simulink model "AttitudeDetermination"  (R2024b)
settings: Solver=VariableStepAuto  StartTime=0.0  StopTime=10.0  RelTol=1e-3
libraries: matrix_library x6
settings Model: Creator=filippocamaleonte  LastModifiedBy=filippocamaleonte

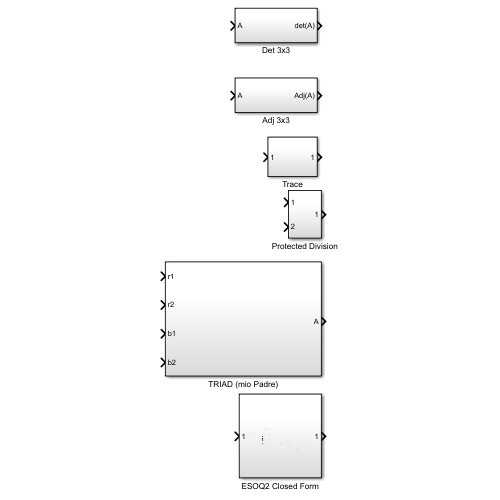
[thumbnail: Simulink's stored preview of the top-level diagram]
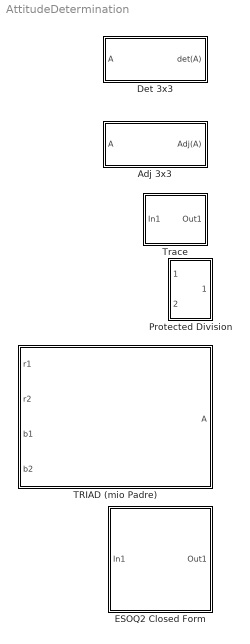
== system AttitudeDetermination ==
  Adj 3x3 : Subsystem
  Det 3x3 : Subsystem
  ESOQ2 Closed Form : Subsystem
  Protected Division : Subsystem
  TRIAD (mio Padre) : Subsystem
  Trace : Subsystem

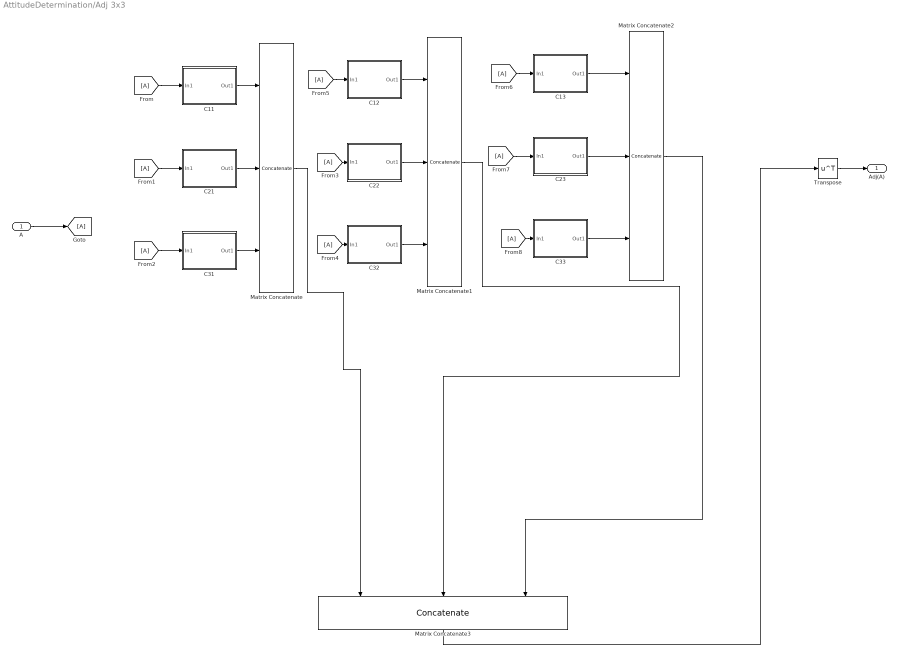
== system AttitudeDetermination/Adj 3x3 ==
  A : Inport
  C11 : Subsystem
  C12 : Subsystem
  C13 : Subsystem
  C21 : Subsystem
  C22 : Subsystem
  C23 : Subsystem
  C31 : Subsystem
  C32 : Subsystem
  C33 : Subsystem
  From{,1..8} (9 alike) : From
  Goto : Goto
  Matrix Concatenate : Concatenate  NumInputs=3  Mode=Multidimensional array
  Matrix Concatenate1 : Concatenate  NumInputs=3  Mode=Multidimensional array
  Matrix Concatenate2 : Concatenate  NumInputs=3  Mode=Multidimensional array
  Matrix Concatenate3 : Concatenate  NumInputs=3  Mode=Multidimensional array  ConcatenateDimension=2
  Transpose : Math  Operator=transpose
  Adj(A) : Outport
  wires:
  Transpose/1 -> Adj(A)/1
  A/1 -> Goto/1
  C11/1(Out1) -> Matrix Concatenate/1
  C21/1(Out1) -> Matrix Concatenate/2
  C31/1(Out1) -> Matrix Concatenate/3
  C22/1(Out1) -> Matrix Concatenate1/2
  C12/1(Out1) -> Matrix Concatenate1/1
  C32/1(Out1) -> Matrix Concatenate1/3
  C23/1(Out1) -> Matrix Concatenate2/2
  C13/1(Out1) -> Matrix Concatenate2/1
  C33/1(Out1) -> Matrix Concatenate2/3
  Matrix Concatenate3/1 -> Transpose/1
  Matrix Concatenate2/1 -> Matrix Concatenate3/3
  Matrix Concatenate1/1 -> Matrix Concatenate3/2
  Matrix Concatenate/1 -> Matrix Concatenate3/1
  From/1 -> C11/1(In1)
  From1/1 -> C21/1(In1)
  From2/1 -> C31/1(In1)
  From3/1 -> C22/1(In1)
  From4/1 -> C32/1(In1)
  From5/1 -> C12/1(In1)
  From6/1 -> C13/1(In1)
  From7/1 -> C23/1(In1)
  From8/1 -> C33/1(In1)

== system AttitudeDetermination/Det 3x3 ==
  A : Inport
  Adj 3x3 : Subsystem
  Matrix Multiply : Product  Multiplication=Matrix(*)
  Selector : Selector  NumberOfDimensions=2  InputPortWidth=3  IndexOptions=Index vector (dialog),Index vector (dialog)  Indices=1,1  OutputSizes=1,1
  det(A) : Outport
  wires:
  A/1 -> Adj 3x3/1(In1), Matrix Multiply/1
  Adj 3x3/1(Out1) -> Matrix Multiply/2
  Matrix Multiply/1 -> Selector/1
  Selector/1 -> det(A)/1

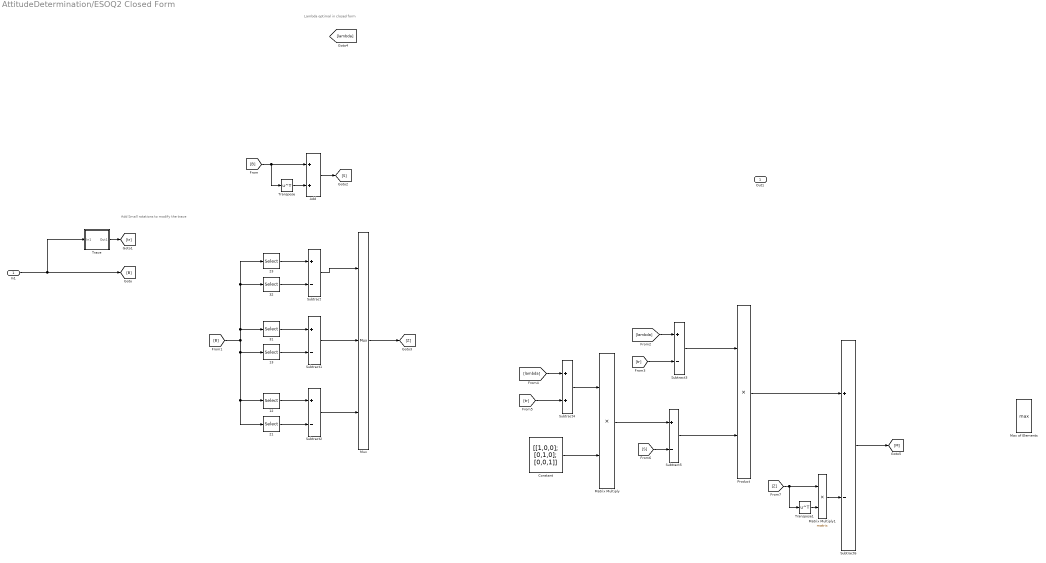
== system AttitudeDetermination/ESOQ2 Closed Form ==
  note: Lambda optimal in closed form
  note: Add Small rotations to modify the trace
  In1 : Inport
  12 : Selector  NumberOfDimensions=2  InputPortWidth=3  IndexOptions=Index vector (dialog),Index vector (dialog)  Indices=1,2  OutputSizes=1,1
  13 : Selector  NumberOfDimensions=2  InputPortWidth=3  IndexOptions=Index vector (dialog),Index vector (dialog)  Indices=1,3  OutputSizes=1,1
  21 : Selector  NumberOfDimensions=2  InputPortWidth=3  IndexOptions=Index vector (dialog),Index vector (dialog)  Indices=2,1  OutputSizes=1,1
  23 : Selector  NumberOfDimensions=2  InputPortWidth=3  IndexOptions=Index vector (dialog),Index vector (dialog)  Indices=2,3  OutputSizes=1,1
  31 : Selector  NumberOfDimensions=2  InputPortWidth=3  IndexOptions=Index vector (dialog),Index vector (dialog)  Indices=3,1  OutputSizes=1,1
  32 : Selector  NumberOfDimensions=2  InputPortWidth=3  IndexOptions=Index vector (dialog),Index vector (dialog)  Indices=3,2  OutputSizes=1,1
  Add : Sum
  Constant : Constant  Value=[[1,0,0]; [0,1,0]; [0,0,1]]
  Matrix Multiply : Product
  Matrix Multiply1 : Product  Multiplication=Matrix(*)
  Max of Elements : MinMax  Function=max
  Mux : Mux  Inputs=3
  Product : Product
  Subtract{,1..3,5..6} (6 alike) : Sum  Inputs=+-
  Subtract4 : Sum
  Trace : Subsystem
  Transpose : Math  Operator=transpose
  Transpose1 : Math  Operator=transpose
  Out1 : Outport
  wires:
  Trace/1(Out1) -> [tr]
  In1/1 -> Trace/1(In1), [B]
  [B] -> Transpose/1, Add/1
  Transpose/1 -> Add/2
  Add/1 -> [S]
  23/1 -> Subtract/1
  32/1 -> Subtract/2
  31/1 -> Subtract1/1
  21/1 -> Subtract2/2
  13/1 -> Subtract1/2
  12/1 -> Subtract2/1
  [B] -> 31/1, 32/1, 23/1, 13/1, 12/1, 21/1
  Subtract1/1 -> Mux/2
  Subtract/1 -> Mux/1
  Subtract2/1 -> Mux/3
  Mux/1 -> [Z]
  [lambda] -> Subtract3/1
  [tr] -> Subtract3/2
  [tr] -> Subtract4/2
  [lambda] -> Subtract4/1
  Subtract4/1 -> Matrix Multiply/1
  Constant/1 -> Matrix Multiply/2
  Matrix Multiply/1 -> Subtract5/1
  [S] -> Subtract5/2
  Product/1 -> Subtract6/1
  Subtract3/1 -> Product/1
  Subtract5/1 -> Product/2
  Matrix Multiply1/1 -> Subtract6/2
  [Z] -> Transpose1/1, Matrix Multiply1/1
  Transpose1/1 -> Matrix Multiply1/2
  Subtract6/1 -> [M]

== system AttitudeDetermination/Protected Division ==
  In1 : Inport
  In2 : Inport  Port=2
  Constant : Constant  Value=eps
  Divide : Product  Inputs=*/
  Switch : Switch  Criteria=u2 ~= 0  SaturateOnIntegerOverflow=off  InputSameDT=off
  Out1 : Outport
  wires:
  Divide/1 -> Out1/1
  In1/1 -> Divide/1
  In2/1 -> Switch/1, Switch/2
  Switch/1 -> Divide/2
  Constant/1 -> Switch/3

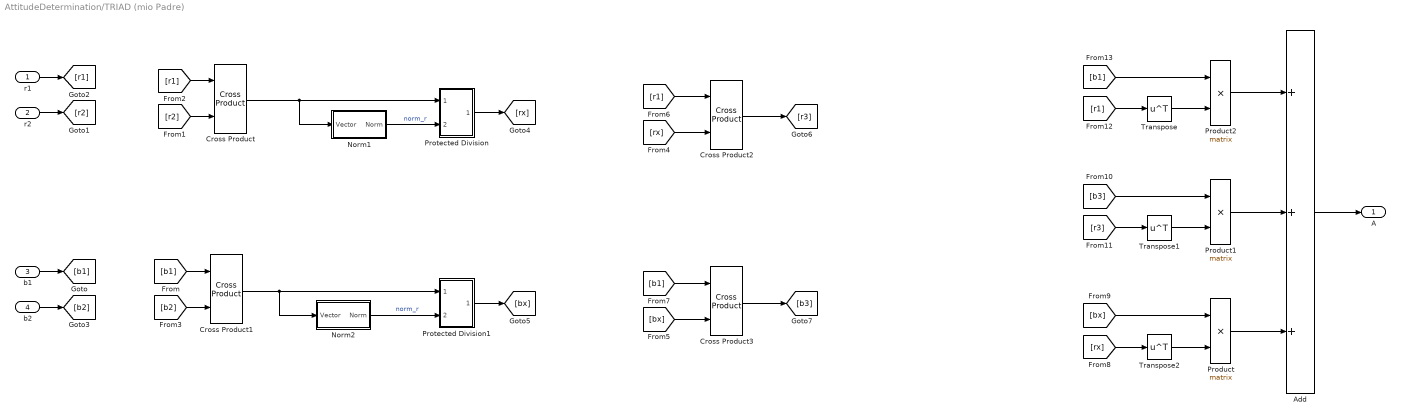
== system AttitudeDetermination/TRIAD (mio Padre) ==
  r1 : Inport
  r2 : Inport  Port=2
  b1 : Inport  Port=3
  b2 : Inport  Port=4
  Add : Sum  Inputs=+++
  Cross Product{,1..3} (4 alike) : matrix_library/Cross Product
  Norm1 : Subsystem
  Norm2 : Subsystem
  Product : Product  Multiplication=Matrix(*)
  Product1 : Product  Multiplication=Matrix(*)
  Product2 : Product  Multiplication=Matrix(*)
  Protected Division : Subsystem
  Protected Division1 : Subsystem
  Transpose : Math  Operator=transpose
  Transpose1 : Math  Operator=transpose
  Transpose2 : Math  Operator=transpose
  A : Outport
  wires:
  Cross Product/1 -> Norm1/1(Vector), Protected Division/1(In1)
  Cross Product1/1 -> Norm2/1(Vector), Protected Division1/1(In1)
  b1/1 -> [b1]
  [b1] -> Cross Product1/1
  r2/1 -> [r2]
  [r2] -> Cross Product/2
  r1/1 -> [r1]
  [r1] -> Cross Product/1
  b2/1 -> [b2]
  [b2] -> Cross Product1/2
  Norm1/1(Norm) -> Protected Division/2(Norm)  "norm_r"
  Norm2/1(Norm) -> Protected Division1/2(Norm)  "norm_r"
  Protected Division/1(Out1) -> [rx]
  Protected Division1/1(Out1) -> [bx]
  [rx] -> Cross Product2/2
  [bx] -> Cross Product3/2
  [r1] -> Cross Product2/1
  [b1] -> Cross Product3/1
  Cross Product2/1 -> [r3]
  Cross Product3/1 -> [b3]
  Add/1 -> A/1
  Product/1 -> Add/3
  Product1/1 -> Add/2
  Product2/1 -> Add/1
  Transpose/1 -> Product2/2
  Transpose1/1 -> Product1/2
  Transpose2/1 -> Product/2
  [rx] -> Transpose2/1
  [bx] -> Product/1
  [b3] -> Product1/1
  [r3] -> Transpose1/1
  [r1] -> Transpose/1
  [b1] -> Product2/1

== system AttitudeDetermination/Trace ==
  In1 : Inport
  Extract Diagonal : matrix_library/Extract Diagonal
      settings: LibrarySourceBlock=|
      | simulink/Matrix
      | Operations/Extract Diagonal
  Sum of Elements : Sum  Inputs=+
  Out1 : Outport
  wires:
  In1/1 -> Extract Diagonal/1
  Extract Diagonal/1 -> Sum of Elements/1
  Sum of Elements/1 -> Out1/1

== system AttitudeDetermination/Adj 3x3/C11 ==
  In1 : Inport
  22 : Selector  NumberOfDimensions=2  InputPortWidth=3  IndexOptions=Index vector (dialog),Index vector (dialog)  Indices=2,2  OutputSizes=1,1
  23 : Selector  NumberOfDimensions=2  InputPortWidth=3  IndexOptions=Index vector (dialog),Index vector (dialog)  Indices=2,3  OutputSizes=1,1
  32 : Selector  NumberOfDimensions=2  InputPortWidth=3  IndexOptions=Index vector (dialog),Index vector (dialog)  Indices=3,2  OutputSizes=1,1
  33 : Selector  NumberOfDimensions=2  InputPortWidth=3  IndexOptions=Index vector (dialog),Index vector (dialog)  Indices=3,3  OutputSizes=1,1
  Product : Product
  Product1 : Product
  Subtract : Sum  Inputs=+-
  Out1 : Outport
  wires:
  In1/1 -> 32/1, 23/1, 33/1, 22/1
  22/1 -> Product/1
  33/1 -> Product/2
  23/1 -> Product1/1
  32/1 -> Product1/2
  Subtract/1 -> Out1/1
  Product/1 -> Subtract/1
  Product1/1 -> Subtract/2

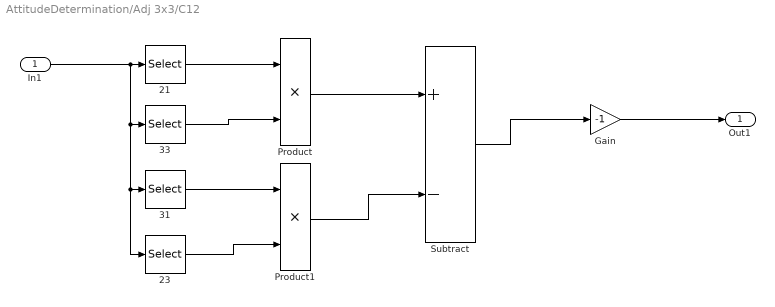
== system AttitudeDetermination/Adj 3x3/C12 ==
  In1 : Inport
  21 : Selector  NumberOfDimensions=2  InputPortWidth=3  IndexOptions=Index vector (dialog),Index vector (dialog)  Indices=2,1  OutputSizes=1,1
  23 : Selector  NumberOfDimensions=2  InputPortWidth=3  IndexOptions=Index vector (dialog),Index vector (dialog)  Indices=2,3  OutputSizes=1,1
  31 : Selector  NumberOfDimensions=2  InputPortWidth=3  IndexOptions=Index vector (dialog),Index vector (dialog)  Indices=3,1  OutputSizes=1,1
  33 : Selector  NumberOfDimensions=2  InputPortWidth=3  IndexOptions=Index vector (dialog),Index vector (dialog)  Indices=3,3  OutputSizes=1,1
  Gain : Gain  Gain=-1
  Product : Product
  Product1 : Product
  Subtract : Sum  Inputs=+-
  Out1 : Outport
  wires:
  In1/1 -> 23/1, 31/1, 33/1, 21/1
  21/1 -> Product/1
  33/1 -> Product/2
  31/1 -> Product1/1
  23/1 -> Product1/2
  Subtract/1 -> Gain/1
  Product/1 -> Subtract/1
  Product1/1 -> Subtract/2
  Gain/1 -> Out1/1

== system AttitudeDetermination/Adj 3x3/C13 ==
  In1 : Inport
  21 : Selector  NumberOfDimensions=2  InputPortWidth=3  IndexOptions=Index vector (dialog),Index vector (dialog)  Indices=2,1  OutputSizes=1,1
  22 : Selector  NumberOfDimensions=2  InputPortWidth=3  IndexOptions=Index vector (dialog),Index vector (dialog)  Indices=2,2  OutputSizes=1,1
  31 : Selector  NumberOfDimensions=2  InputPortWidth=3  IndexOptions=Index vector (dialog),Index vector (dialog)  Indices=3,1  OutputSizes=1,1
  32 : Selector  NumberOfDimensions=2  InputPortWidth=3  IndexOptions=Index vector (dialog),Index vector (dialog)  Indices=3,2  OutputSizes=1,1
  Product : Product
  Product1 : Product
  Subtract : Sum  Inputs=+-
  Out1 : Outport
  wires:
  In1/1 -> 31/1, 22/1, 32/1, 21/1
  21/1 -> Product/1
  32/1 -> Product/2
  22/1 -> Product1/1
  31/1 -> Product1/2
  Subtract/1 -> Out1/1
  Product/1 -> Subtract/1
  Product1/1 -> Subtract/2

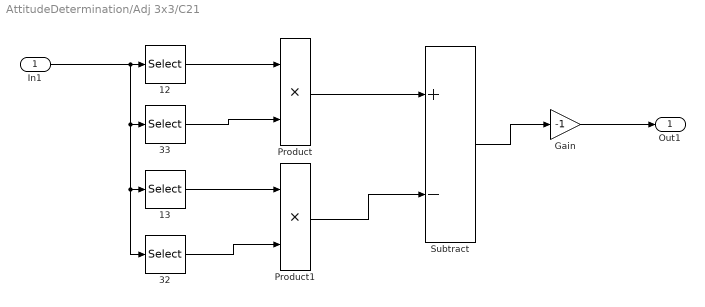
== system AttitudeDetermination/Adj 3x3/C21 ==
  In1 : Inport
  12 : Selector  NumberOfDimensions=2  InputPortWidth=3  IndexOptions=Index vector (dialog),Index vector (dialog)  Indices=1,2  OutputSizes=1,1
  13 : Selector  NumberOfDimensions=2  InputPortWidth=3  IndexOptions=Index vector (dialog),Index vector (dialog)  Indices=1,3  OutputSizes=1,1
  32 : Selector  NumberOfDimensions=2  InputPortWidth=3  IndexOptions=Index vector (dialog),Index vector (dialog)  Indices=3,2  OutputSizes=1,1
  33 : Selector  NumberOfDimensions=2  InputPortWidth=3  IndexOptions=Index vector (dialog),Index vector (dialog)  Indices=3,3  OutputSizes=1,1
  Gain : Gain  Gain=-1
  Product : Product
  Product1 : Product
  Subtract : Sum  Inputs=+-
  Out1 : Outport
  wires:
  In1/1 -> 32/1, 13/1, 33/1, 12/1
  12/1 -> Product/1
  33/1 -> Product/2
  13/1 -> Product1/1
  32/1 -> Product1/2
  Subtract/1 -> Gain/1
  Product/1 -> Subtract/1
  Product1/1 -> Subtract/2
  Gain/1 -> Out1/1

== system AttitudeDetermination/Adj 3x3/C22 ==
  In1 : Inport
  11 : Selector  NumberOfDimensions=2  InputPortWidth=3  IndexOptions=Index vector (dialog),Index vector (dialog)  Indices=1,1  OutputSizes=1,1
  13 : Selector  NumberOfDimensions=2  InputPortWidth=3  IndexOptions=Index vector (dialog),Index vector (dialog)  Indices=1,3  OutputSizes=1,1
  31 : Selector  NumberOfDimensions=2  InputPortWidth=3  IndexOptions=Index vector (dialog),Index vector (dialog)  Indices=3,1  OutputSizes=1,1
  33 : Selector  NumberOfDimensions=2  InputPortWidth=3  IndexOptions=Index vector (dialog),Index vector (dialog)  Indices=3,3  OutputSizes=1,1
  Product : Product
  Product1 : Product
  Subtract : Sum  Inputs=+-
  Out1 : Outport
  wires:
  In1/1 -> 31/1, 13/1, 33/1, 11/1
  11/1 -> Product/1
  33/1 -> Product/2
  13/1 -> Product1/1
  31/1 -> Product1/2
  Subtract/1 -> Out1/1
  Product/1 -> Subtract/1
  Product1/1 -> Subtract/2

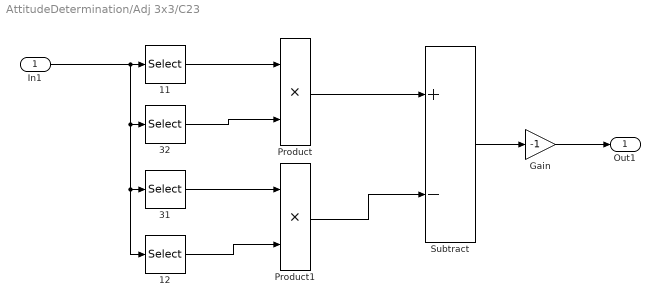
== system AttitudeDetermination/Adj 3x3/C23 ==
  In1 : Inport
  11 : Selector  NumberOfDimensions=2  InputPortWidth=3  IndexOptions=Index vector (dialog),Index vector (dialog)  Indices=1,1  OutputSizes=1,1
  12 : Selector  NumberOfDimensions=2  InputPortWidth=3  IndexOptions=Index vector (dialog),Index vector (dialog)  Indices=1,2  OutputSizes=1,1
  31 : Selector  NumberOfDimensions=2  InputPortWidth=3  IndexOptions=Index vector (dialog),Index vector (dialog)  Indices=3,1  OutputSizes=1,1
  32 : Selector  NumberOfDimensions=2  InputPortWidth=3  IndexOptions=Index vector (dialog),Index vector (dialog)  Indices=3,2  OutputSizes=1,1
  Gain : Gain  Gain=-1
  Product : Product
  Product1 : Product
  Subtract : Sum  Inputs=+-
  Out1 : Outport
  wires:
  In1/1 -> 12/1, 31/1, 32/1, 11/1
  11/1 -> Product/1
  32/1 -> Product/2
  31/1 -> Product1/1
  12/1 -> Product1/2
  Subtract/1 -> Gain/1
  Product/1 -> Subtract/1
  Product1/1 -> Subtract/2
  Gain/1 -> Out1/1

== system AttitudeDetermination/Adj 3x3/C31 ==
  In1 : Inport
  12 : Selector  NumberOfDimensions=2  InputPortWidth=3  IndexOptions=Index vector (dialog),Index vector (dialog)  Indices=1,2  OutputSizes=1,1
  13 : Selector  NumberOfDimensions=2  InputPortWidth=3  IndexOptions=Index vector (dialog),Index vector (dialog)  Indices=1,3  OutputSizes=1,1
  22 : Selector  NumberOfDimensions=2  InputPortWidth=3  IndexOptions=Index vector (dialog),Index vector (dialog)  Indices=2,2  OutputSizes=1,1
  23 : Selector  NumberOfDimensions=2  InputPortWidth=3  IndexOptions=Index vector (dialog),Index vector (dialog)  Indices=2,3  OutputSizes=1,1
  Product : Product
  Product1 : Product
  Subtract : Sum  Inputs=+-
  Out1 : Outport
  wires:
  In1/1 -> 22/1, 13/1, 23/1, 12/1
  12/1 -> Product/1
  23/1 -> Product/2
  13/1 -> Product1/1
  22/1 -> Product1/2
  Subtract/1 -> Out1/1
  Product/1 -> Subtract/1
  Product1/1 -> Subtract/2

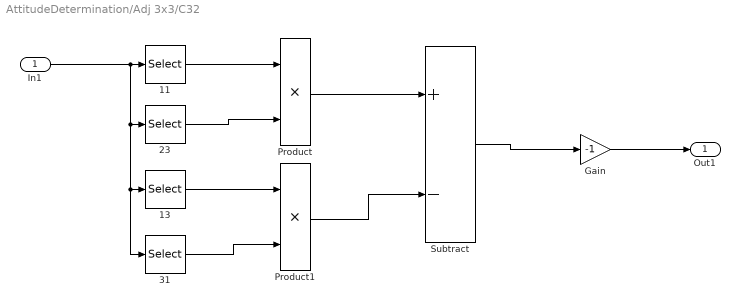
== system AttitudeDetermination/Adj 3x3/C32 ==
  In1 : Inport
  11 : Selector  NumberOfDimensions=2  InputPortWidth=3  IndexOptions=Index vector (dialog),Index vector (dialog)  Indices=1,1  OutputSizes=1,1
  13 : Selector  NumberOfDimensions=2  InputPortWidth=3  IndexOptions=Index vector (dialog),Index vector (dialog)  Indices=1,3  OutputSizes=1,1
  23 : Selector  NumberOfDimensions=2  InputPortWidth=3  IndexOptions=Index vector (dialog),Index vector (dialog)  Indices=2,3  OutputSizes=1,1
  31 : Selector  NumberOfDimensions=2  InputPortWidth=3  IndexOptions=Index vector (dialog),Index vector (dialog)  Indices=3,1  OutputSizes=1,1
  Gain : Gain  Gain=-1
  Product : Product
  Product1 : Product
  Subtract : Sum  Inputs=+-
  Out1 : Outport
  wires:
  In1/1 -> 31/1, 13/1, 23/1, 11/1
  11/1 -> Product/1
  23/1 -> Product/2
  13/1 -> Product1/1
  31/1 -> Product1/2
  Subtract/1 -> Gain/1
  Product/1 -> Subtract/1
  Product1/1 -> Subtract/2
  Gain/1 -> Out1/1

== system AttitudeDetermination/Adj 3x3/C33 ==
  In1 : Inport
  11 : Selector  NumberOfDimensions=2  InputPortWidth=3  IndexOptions=Index vector (dialog),Index vector (dialog)  Indices=1,1  OutputSizes=1,1
  12 : Selector  NumberOfDimensions=2  InputPortWidth=3  IndexOptions=Index vector (dialog),Index vector (dialog)  Indices=1,2  OutputSizes=1,1
  21 : Selector  NumberOfDimensions=2  InputPortWidth=3  IndexOptions=Index vector (dialog),Index vector (dialog)  Indices=2,1  OutputSizes=1,1
  22 : Selector  NumberOfDimensions=2  InputPortWidth=3  IndexOptions=Index vector (dialog),Index vector (dialog)  Indices=2,2  OutputSizes=1,1
  Product : Product
  Product1 : Product
  Subtract : Sum  Inputs=+-
  Out1 : Outport
  wires:
  In1/1 -> 21/1, 12/1, 22/1, 11/1
  11/1 -> Product/1
  22/1 -> Product/2
  12/1 -> Product1/1
  21/1 -> Product1/2
  Subtract/1 -> Out1/1
  Product/1 -> Subtract/1
  Product1/1 -> Subtract/2

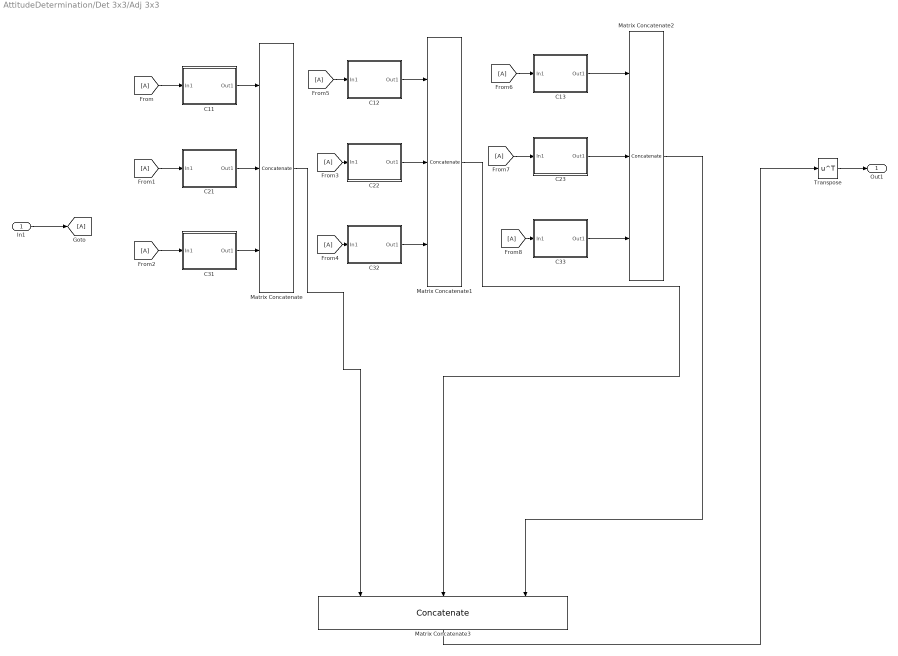
== system AttitudeDetermination/Det 3x3/Adj 3x3 ==
  In1 : Inport
  C11 : Subsystem
  C12 : Subsystem
  C13 : Subsystem
  C21 : Subsystem
  C22 : Subsystem
  C23 : Subsystem
  C31 : Subsystem
  C32 : Subsystem
  C33 : Subsystem
  From{,1..8} (9 alike) : From
  Goto : Goto
  Matrix Concatenate : Concatenate  NumInputs=3  Mode=Multidimensional array
  Matrix Concatenate1 : Concatenate  NumInputs=3  Mode=Multidimensional array
  Matrix Concatenate2 : Concatenate  NumInputs=3  Mode=Multidimensional array
  Matrix Concatenate3 : Concatenate  NumInputs=3  Mode=Multidimensional array  ConcatenateDimension=2
  Transpose : Math  Operator=transpose
  Out1 : Outport
  wires:
  Transpose/1 -> Out1/1
  In1/1 -> Goto/1
  C11/1(Out1) -> Matrix Concatenate/1
  C21/1(Out1) -> Matrix Concatenate/2
  C31/1(Out1) -> Matrix Concatenate/3
  C22/1(Out1) -> Matrix Concatenate1/2
  C12/1(Out1) -> Matrix Concatenate1/1
  C32/1(Out1) -> Matrix Concatenate1/3
  C23/1(Out1) -> Matrix Concatenate2/2
  C13/1(Out1) -> Matrix Concatenate2/1
  C33/1(Out1) -> Matrix Concatenate2/3
  Matrix Concatenate3/1 -> Transpose/1
  Matrix Concatenate2/1 -> Matrix Concatenate3/3
  Matrix Concatenate1/1 -> Matrix Concatenate3/2
  Matrix Concatenate/1 -> Matrix Concatenate3/1
  From/1 -> C11/1(In1)
  From1/1 -> C21/1(In1)
  From2/1 -> C31/1(In1)
  From3/1 -> C22/1(In1)
  From4/1 -> C32/1(In1)
  From5/1 -> C12/1(In1)
  From6/1 -> C13/1(In1)
  From7/1 -> C23/1(In1)
  From8/1 -> C33/1(In1)

== system AttitudeDetermination/ESOQ2 Closed Form/Trace ==
  In1 : Inport
  Extract Diagonal : matrix_library/Extract Diagonal
  Sum of Elements : Sum  Inputs=+
  Out1 : Outport
  wires:
  In1/1 -> Extract Diagonal/1
  Extract Diagonal/1 -> Sum of Elements/1
  Sum of Elements/1 -> Out1/1

== system AttitudeDetermination/TRIAD (mio Padre)/Norm1 ==
  Vector : Inport
  Add : Sum  Inputs=+++
  Demux : Demux  Outputs=3
  Sqrt : Sqrt
  Square : Math  Operator=square
  Square1 : Math  Operator=square
  Square2 : Math  Operator=square
  Norm : Outport
  wires:
  Square/1 -> Add/1
  Add/1 -> Sqrt/1
  Demux/3 -> Square1/1
  Square2/1 -> Add/2
  Square1/1 -> Add/3
  Demux/1 -> Square/1
  Demux/2 -> Square2/1
  Vector/1 -> Demux/1
  Sqrt/1 -> Norm/1

== system AttitudeDetermination/TRIAD (mio Padre)/Norm2 ==
  Vector : Inport
  Add : Sum  Inputs=+++
  Demux : Demux  Outputs=3
  Sqrt : Sqrt
  Square : Math  Operator=square
  Square1 : Math  Operator=square
  Square2 : Math  Operator=square
  Norm : Outport
  wires:
  Square/1 -> Add/1
  Add/1 -> Sqrt/1
  Demux/3 -> Square1/1
  Square2/1 -> Add/2
  Square1/1 -> Add/3
  Demux/1 -> Square/1
  Demux/2 -> Square2/1
  Vector/1 -> Demux/1
  Sqrt/1 -> Norm/1

== system AttitudeDetermination/TRIAD (mio Padre)/Protected Division ==
  In1 : Inport
  Norm : Inport  Port=2
  Constant : Constant  Value=eps
  Divide : Product  Inputs=*/
  Switch : Switch  Criteria=u2 ~= 0  SaturateOnIntegerOverflow=off  InputSameDT=off
  Out1 : Outport
  wires:
  Divide/1 -> Out1/1
  In1/1 -> Divide/1
  Norm/1 -> Switch/1, Switch/2
  Switch/1 -> Divide/2
  Constant/1 -> Switch/3

== system AttitudeDetermination/TRIAD (mio Padre)/Protected Division1 ==
  In1 : Inport
  Norm : Inport  Port=2
  Constant : Constant  Value=eps
  Divide : Product  Inputs=*/
  Switch : Switch  Criteria=u2 ~= 0  SaturateOnIntegerOverflow=off  InputSameDT=off
  Out1 : Outport
  wires:
  Divide/1 -> Out1/1
  In1/1 -> Divide/1
  Norm/1 -> Switch/1, Switch/2
  Switch/1 -> Divide/2
  Constant/1 -> Switch/3

== system AttitudeDetermination/Det 3x3/Adj 3x3/C11 ==
  In1 : Inport
  22 : Selector  NumberOfDimensions=2  InputPortWidth=3  IndexOptions=Index vector (dialog),Index vector (dialog)  Indices=2,2  OutputSizes=1,1
  23 : Selector  NumberOfDimensions=2  InputPortWidth=3  IndexOptions=Index vector (dialog),Index vector (dialog)  Indices=2,3  OutputSizes=1,1
  32 : Selector  NumberOfDimensions=2  InputPortWidth=3  IndexOptions=Index vector (dialog),Index vector (dialog)  Indices=3,2  OutputSizes=1,1
  33 : Selector  NumberOfDimensions=2  InputPortWidth=3  IndexOptions=Index vector (dialog),Index vector (dialog)  Indices=3,3  OutputSizes=1,1
  Product : Product
  Product1 : Product
  Subtract : Sum  Inputs=+-
  Out1 : Outport
  wires:
  In1/1 -> 32/1, 23/1, 33/1, 22/1
  22/1 -> Product/1
  33/1 -> Product/2
  23/1 -> Product1/1
  32/1 -> Product1/2
  Subtract/1 -> Out1/1
  Product/1 -> Subtract/1
  Product1/1 -> Subtract/2

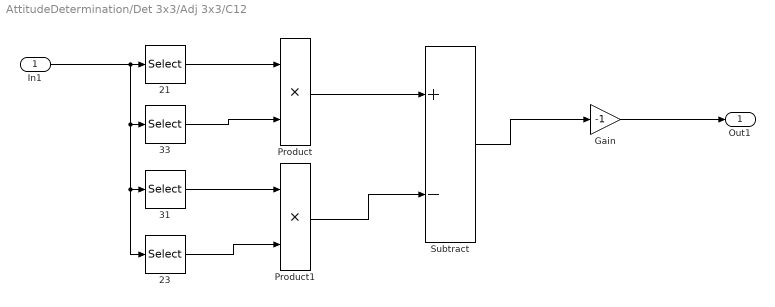
== system AttitudeDetermination/Det 3x3/Adj 3x3/C12 ==
  In1 : Inport
  21 : Selector  NumberOfDimensions=2  InputPortWidth=3  IndexOptions=Index vector (dialog),Index vector (dialog)  Indices=2,1  OutputSizes=1,1
  23 : Selector  NumberOfDimensions=2  InputPortWidth=3  IndexOptions=Index vector (dialog),Index vector (dialog)  Indices=2,3  OutputSizes=1,1
  31 : Selector  NumberOfDimensions=2  InputPortWidth=3  IndexOptions=Index vector (dialog),Index vector (dialog)  Indices=3,1  OutputSizes=1,1
  33 : Selector  NumberOfDimensions=2  InputPortWidth=3  IndexOptions=Index vector (dialog),Index vector (dialog)  Indices=3,3  OutputSizes=1,1
  Gain : Gain  Gain=-1
  Product : Product
  Product1 : Product
  Subtract : Sum  Inputs=+-
  Out1 : Outport
  wires:
  In1/1 -> 23/1, 31/1, 33/1, 21/1
  21/1 -> Product/1
  33/1 -> Product/2
  31/1 -> Product1/1
  23/1 -> Product1/2
  Subtract/1 -> Gain/1
  Product/1 -> Subtract/1
  Product1/1 -> Subtract/2
  Gain/1 -> Out1/1

== system AttitudeDetermination/Det 3x3/Adj 3x3/C13 ==
  In1 : Inport
  21 : Selector  NumberOfDimensions=2  InputPortWidth=3  IndexOptions=Index vector (dialog),Index vector (dialog)  Indices=2,1  OutputSizes=1,1
  22 : Selector  NumberOfDimensions=2  InputPortWidth=3  IndexOptions=Index vector (dialog),Index vector (dialog)  Indices=2,2  OutputSizes=1,1
  31 : Selector  NumberOfDimensions=2  InputPortWidth=3  IndexOptions=Index vector (dialog),Index vector (dialog)  Indices=3,1  OutputSizes=1,1
  32 : Selector  NumberOfDimensions=2  InputPortWidth=3  IndexOptions=Index vector (dialog),Index vector (dialog)  Indices=3,2  OutputSizes=1,1
  Product : Product
  Product1 : Product
  Subtract : Sum  Inputs=+-
  Out1 : Outport
  wires:
  In1/1 -> 31/1, 22/1, 32/1, 21/1
  21/1 -> Product/1
  32/1 -> Product/2
  22/1 -> Product1/1
  31/1 -> Product1/2
  Subtract/1 -> Out1/1
  Product/1 -> Subtract/1
  Product1/1 -> Subtract/2

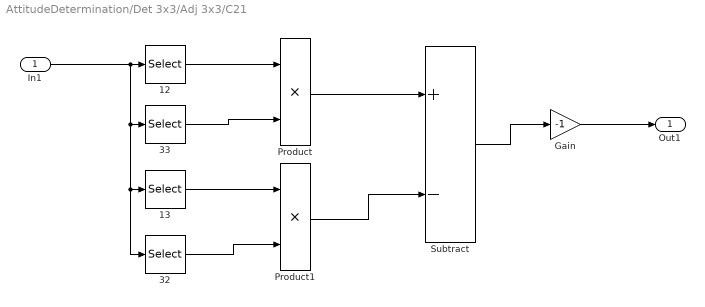
== system AttitudeDetermination/Det 3x3/Adj 3x3/C21 ==
  In1 : Inport
  12 : Selector  NumberOfDimensions=2  InputPortWidth=3  IndexOptions=Index vector (dialog),Index vector (dialog)  Indices=1,2  OutputSizes=1,1
  13 : Selector  NumberOfDimensions=2  InputPortWidth=3  IndexOptions=Index vector (dialog),Index vector (dialog)  Indices=1,3  OutputSizes=1,1
  32 : Selector  NumberOfDimensions=2  InputPortWidth=3  IndexOptions=Index vector (dialog),Index vector (dialog)  Indices=3,2  OutputSizes=1,1
  33 : Selector  NumberOfDimensions=2  InputPortWidth=3  IndexOptions=Index vector (dialog),Index vector (dialog)  Indices=3,3  OutputSizes=1,1
  Gain : Gain  Gain=-1
  Product : Product
  Product1 : Product
  Subtract : Sum  Inputs=+-
  Out1 : Outport
  wires:
  In1/1 -> 32/1, 13/1, 33/1, 12/1
  12/1 -> Product/1
  33/1 -> Product/2
  13/1 -> Product1/1
  32/1 -> Product1/2
  Subtract/1 -> Gain/1
  Product/1 -> Subtract/1
  Product1/1 -> Subtract/2
  Gain/1 -> Out1/1

== system AttitudeDetermination/Det 3x3/Adj 3x3/C22 ==
  In1 : Inport
  11 : Selector  NumberOfDimensions=2  InputPortWidth=3  IndexOptions=Index vector (dialog),Index vector (dialog)  Indices=1,1  OutputSizes=1,1
  13 : Selector  NumberOfDimensions=2  InputPortWidth=3  IndexOptions=Index vector (dialog),Index vector (dialog)  Indices=1,3  OutputSizes=1,1
  31 : Selector  NumberOfDimensions=2  InputPortWidth=3  IndexOptions=Index vector (dialog),Index vector (dialog)  Indices=3,1  OutputSizes=1,1
  33 : Selector  NumberOfDimensions=2  InputPortWidth=3  IndexOptions=Index vector (dialog),Index vector (dialog)  Indices=3,3  OutputSizes=1,1
  Product : Product
  Product1 : Product
  Subtract : Sum  Inputs=+-
  Out1 : Outport
  wires:
  In1/1 -> 31/1, 13/1, 33/1, 11/1
  11/1 -> Product/1
  33/1 -> Product/2
  13/1 -> Product1/1
  31/1 -> Product1/2
  Subtract/1 -> Out1/1
  Product/1 -> Subtract/1
  Product1/1 -> Subtract/2

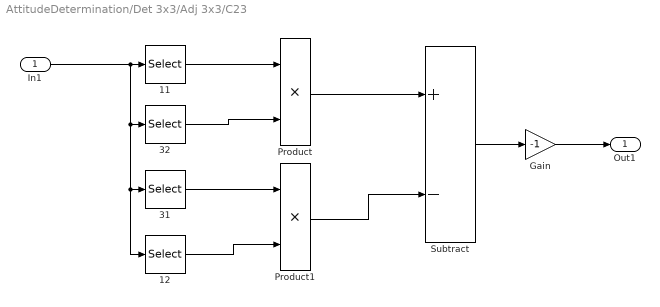
== system AttitudeDetermination/Det 3x3/Adj 3x3/C23 ==
  In1 : Inport
  11 : Selector  NumberOfDimensions=2  InputPortWidth=3  IndexOptions=Index vector (dialog),Index vector (dialog)  Indices=1,1  OutputSizes=1,1
  12 : Selector  NumberOfDimensions=2  InputPortWidth=3  IndexOptions=Index vector (dialog),Index vector (dialog)  Indices=1,2  OutputSizes=1,1
  31 : Selector  NumberOfDimensions=2  InputPortWidth=3  IndexOptions=Index vector (dialog),Index vector (dialog)  Indices=3,1  OutputSizes=1,1
  32 : Selector  NumberOfDimensions=2  InputPortWidth=3  IndexOptions=Index vector (dialog),Index vector (dialog)  Indices=3,2  OutputSizes=1,1
  Gain : Gain  Gain=-1
  Product : Product
  Product1 : Product
  Subtract : Sum  Inputs=+-
  Out1 : Outport
  wires:
  In1/1 -> 12/1, 31/1, 32/1, 11/1
  11/1 -> Product/1
  32/1 -> Product/2
  31/1 -> Product1/1
  12/1 -> Product1/2
  Subtract/1 -> Gain/1
  Product/1 -> Subtract/1
  Product1/1 -> Subtract/2
  Gain/1 -> Out1/1

== system AttitudeDetermination/Det 3x3/Adj 3x3/C31 ==
  In1 : Inport
  12 : Selector  NumberOfDimensions=2  InputPortWidth=3  IndexOptions=Index vector (dialog),Index vector (dialog)  Indices=1,2  OutputSizes=1,1
  13 : Selector  NumberOfDimensions=2  InputPortWidth=3  IndexOptions=Index vector (dialog),Index vector (dialog)  Indices=1,3  OutputSizes=1,1
  22 : Selector  NumberOfDimensions=2  InputPortWidth=3  IndexOptions=Index vector (dialog),Index vector (dialog)  Indices=2,2  OutputSizes=1,1
  23 : Selector  NumberOfDimensions=2  InputPortWidth=3  IndexOptions=Index vector (dialog),Index vector (dialog)  Indices=2,3  OutputSizes=1,1
  Product : Product
  Product1 : Product
  Subtract : Sum  Inputs=+-
  Out1 : Outport
  wires:
  In1/1 -> 22/1, 13/1, 23/1, 12/1
  12/1 -> Product/1
  23/1 -> Product/2
  13/1 -> Product1/1
  22/1 -> Product1/2
  Subtract/1 -> Out1/1
  Product/1 -> Subtract/1
  Product1/1 -> Subtract/2

== system AttitudeDetermination/Det 3x3/Adj 3x3/C32 ==
  In1 : Inport
  11 : Selector  NumberOfDimensions=2  InputPortWidth=3  IndexOptions=Index vector (dialog),Index vector (dialog)  Indices=1,1  OutputSizes=1,1
  13 : Selector  NumberOfDimensions=2  InputPortWidth=3  IndexOptions=Index vector (dialog),Index vector (dialog)  Indices=1,3  OutputSizes=1,1
  23 : Selector  NumberOfDimensions=2  InputPortWidth=3  IndexOptions=Index vector (dialog),Index vector (dialog)  Indices=2,3  OutputSizes=1,1
  31 : Selector  NumberOfDimensions=2  InputPortWidth=3  IndexOptions=Index vector (dialog),Index vector (dialog)  Indices=3,1  OutputSizes=1,1
  Gain : Gain  Gain=-1
  Product : Product
  Product1 : Product
  Subtract : Sum  Inputs=+-
  Out1 : Outport
  wires:
  In1/1 -> 31/1, 13/1, 23/1, 11/1
  11/1 -> Product/1
  23/1 -> Product/2
  13/1 -> Product1/1
  31/1 -> Product1/2
  Subtract/1 -> Gain/1
  Product/1 -> Subtract/1
  Product1/1 -> Subtract/2
  Gain/1 -> Out1/1

== system AttitudeDetermination/Det 3x3/Adj 3x3/C33 ==
  In1 : Inport
  11 : Selector  NumberOfDimensions=2  InputPortWidth=3  IndexOptions=Index vector (dialog),Index vector (dialog)  Indices=1,1  OutputSizes=1,1
  12 : Selector  NumberOfDimensions=2  InputPortWidth=3  IndexOptions=Index vector (dialog),Index vector (dialog)  Indices=1,2  OutputSizes=1,1
  21 : Selector  NumberOfDimensions=2  InputPortWidth=3  IndexOptions=Index vector (dialog),Index vector (dialog)  Indices=2,1  OutputSizes=1,1
  22 : Selector  NumberOfDimensions=2  InputPortWidth=3  IndexOptions=Index vector (dialog),Index vector (dialog)  Indices=2,2  OutputSizes=1,1
  Product : Product
  Product1 : Product
  Subtract : Sum  Inputs=+-
  Out1 : Outport
  wires:
  In1/1 -> 21/1, 12/1, 22/1, 11/1
  11/1 -> Product/1
  22/1 -> Product/2
  12/1 -> Product1/1
  21/1 -> Product1/2
  Subtract/1 -> Out1/1
  Product/1 -> Subtract/1
  Product1/1 -> Subtract/2
